simulink model "exp5_diagrama"  (R2020b)
settings: Solver=VariableStepAuto  StartTime=0.0  StopTime=5  RelTol=1e-3
values from neighbouring files (symbols this model uses):
  h = 1e-3    (= 0.001)    [exp5_script.m]
  Kp = (2*zeta*wn*tau-1)/K    [exp5_script.m]
  R_finalvalue = 5    [exp5_script.m]
  R_initialvalue = 3    [exp5_script.m]
  R_steptime = 1    [exp5_script.m]
  Ti = 1/Fi    [exp5_script.m]
undefined symbols (not defined in the file or in its folder): A, B, C, Kt
libraries: simulink x4
settings Model: Creator=lucas  LastModifiedBy=lucas

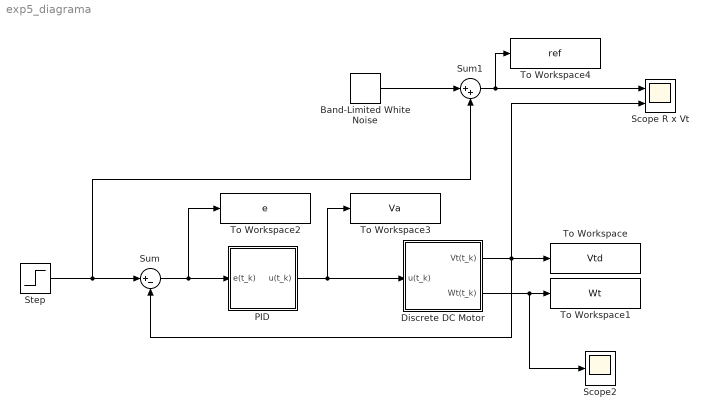
== system exp5_diagrama ==
  Band-Limited White Noise : simulink/Sources/Band-Limited White Noise  Cov=[0.000001]  Ts=0.001  seed=[23341]
  Discrete DC Motor : Subsystem
  PID : Subsystem
  Scope R x Vt : Scope  NumInputPorts=2
  Scope2 : Scope
  Step : Step  Time=R_steptime  Before=R_initialvalue  After=R_finalvalue  SampleTime=h*0.99  VectorParams1D=off  ZeroCross=off
  Sum : Sum  Inputs=|+-
  Sum1 : Sum  Inputs=|++
  To Workspace : ToWorkspace  VariableName=Vtd  SaveFormat=Structure With Time  SampleTime=-1
  To Workspace1 : ToWorkspace  VariableName=Wt  SaveFormat=Structure With Time  SampleTime=-1
  To Workspace2 : ToWorkspace  VariableName=e  SaveFormat=Structure With Time  SampleTime=-1
  To Workspace3 : ToWorkspace  VariableName=Va  SaveFormat=Structure With Time  SampleTime=-1
  To Workspace4 : ToWorkspace  VariableName=ref  SaveFormat=Structure With Time  SampleTime=-1
  wires:
  Step/1 -> Sum1/2, Sum/1
  Band-Limited White Noise/1 -> Sum1/1
  Sum/1 -> To Workspace2/1, PID/1(e(t_k))
  PID/1(u(t_k)) -> To Workspace3/1, Discrete DC Motor/1(u(t_k))
  Sum1/1 -> To Workspace4/1, Scope R x Vt/1
  Discrete DC Motor/1(Vt(t_k)) -> Sum/2, To Workspace/1, Scope R x Vt/2
  Discrete DC Motor/2(Wt(t_k)) -> Scope2/1, To Workspace1/1

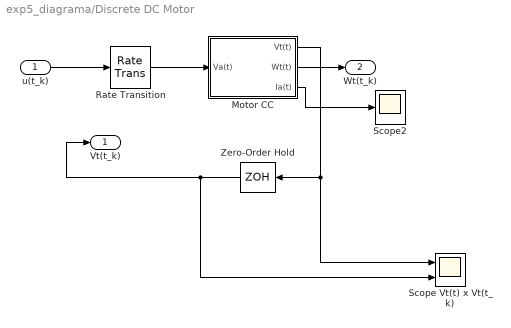
== system exp5_diagrama/Discrete DC Motor ==
  u(t_k) : Inport
  Motor CC : Subsystem
  Rate Transition : RateTransition  OutPortSampleTime=h_motor
  Scope Vt(t) x Vt(t_k) : Scope  NumInputPorts=2
  Scope2 : Scope
  Zero-Order Hold : ZeroOrderHold  SampleTime=h
  Vt(t_k) : Outport
  Wt(t_k) : Outport  Port=2
  wires:
  u(t_k)/1 -> Rate Transition/1
  Zero-Order Hold/1 -> Vt(t_k)/1, Scope Vt(t) x Vt(t_k)/2
  Rate Transition/1 -> Motor CC/1(Va(t))
  Motor CC/1(Vt(t)) -> Scope Vt(t) x Vt(t_k)/1, Zero-Order Hold/1
  Motor CC/3(Ia(t)) -> Scope2/1
  Motor CC/2(Wt(t)) -> Wt(t_k)/1

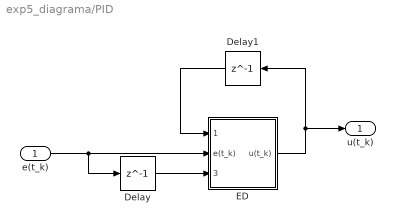
== system exp5_diagrama/PID ==
  e(t_k) : Inport
  Delay : Delay  DelayLength=1
  Delay1 : Delay  DelayLength=1  InitialCondition=0
  ED : Subsystem
  u(t_k) : Outport
  wires:
  Delay/1 -> ED/3(e(t_k-1))
  e(t_k)/1 -> ED/2(e(t_k)), Delay/1
  ED/1(u(t_k)) -> u(t_k)/1, Delay1/1
  Delay1/1 -> ED/1(u(t_k-1))

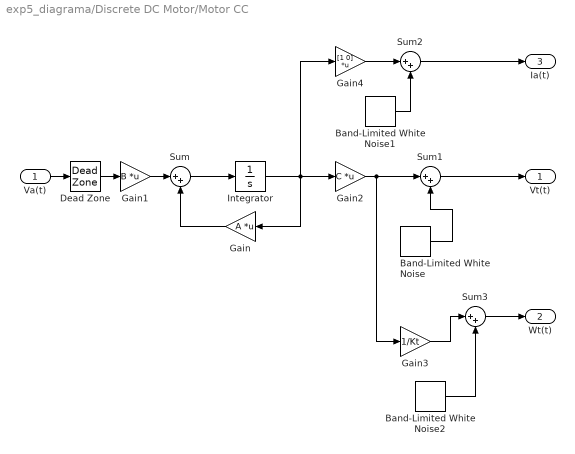
== system exp5_diagrama/Discrete DC Motor/Motor CC ==
  Va(t) : Inport
  Band-Limited White Noise : simulink/Sources/Band-Limited White Noise  Cov=[0.000005]  Ts=0.001  seed=[23341]
  Band-Limited White Noise1 : simulink/Sources/Band-Limited White Noise  Cov=[0.00000001]  Ts=0.001  seed=[23341]
  Band-Limited White Noise2 : simulink/Sources/Band-Limited White Noise  Cov=[0.0007]  Ts=0.001  seed=[23341]
  Dead Zone : DeadZone  LowerValue=-3.2  UpperValue=3.2  SaturateOnIntegerOverflow=on
  Gain : Gain  Gain=A  Multiplication=Matrix(K*u)
  Gain1 : Gain  Gain=B  Multiplication=Matrix(K*u)
  Gain2 : Gain  Gain=C  Multiplication=Matrix(K*u)
  Gain3 : Gain  Gain=1/Kt
  Gain4 : Gain  Gain=[1 0]  Multiplication=Matrix(K*u)
  Integrator : Integrator
  Sum{,1..3} (4 alike) : Sum  Inputs=|++
  Vt(t) : Outport
  Wt(t) : Outport  Port=2
  Ia(t) : Outport  Port=3
  wires:
  Sum/1 -> Integrator/1
  Integrator/1 -> Gain4/1, Gain2/1, Gain/1
  Gain2/1 -> Sum1/1, Gain3/1
  Gain1/1 -> Sum/1
  Gain/1 -> Sum/2
  Va(t)/1 -> Dead Zone/1
  Dead Zone/1 -> Gain1/1
  Sum1/1 -> Vt(t)/1
  Band-Limited White Noise/1 -> Sum1/2
  Sum2/1 -> Ia(t)/1
  Gain4/1 -> Sum2/1
  Sum3/1 -> Wt(t)/1
  Band-Limited White Noise1/1 -> Sum2/2
  Band-Limited White Noise2/1 -> Sum3/2
  Gain3/1 -> Sum3/1

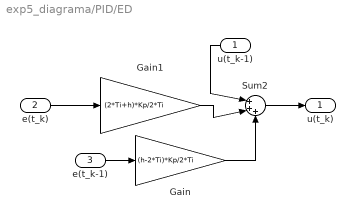
== system exp5_diagrama/PID/ED ==
  u(t_k-1) : Inport
  e(t_k) : Inport  Port=2
  e(t_k-1) : Inport  Port=3
  Gain : Gain  Gain=(h-2*Ti)*Kp/2*Ti
  Gain1 : Gain  Gain=(2*Ti+h)*Kp/2*Ti
  Sum2 : Sum  Inputs=|+++
  u(t_k) : Outport
  wires:
  e(t_k)/1 -> Gain1/1
  Gain1/1 -> Sum2/2
  Sum2/1 -> u(t_k)/1
  Gain/1 -> Sum2/3
  e(t_k-1)/1 -> Gain/1
  u(t_k-1)/1 -> Sum2/1
